simulink model "shafExPosSys"  (R2014a)
settings: Solver=ode3  StartTime=0.0  StopTime=TSIM  FixedStep=1/10  RelTol=1e-3
undefined symbols (not defined in the file): B, C, d, F, H, K, T, x1_0, x2_0, x3_0
settings Model: Creator=sqn4594  LastModifiedBy=sqn4594

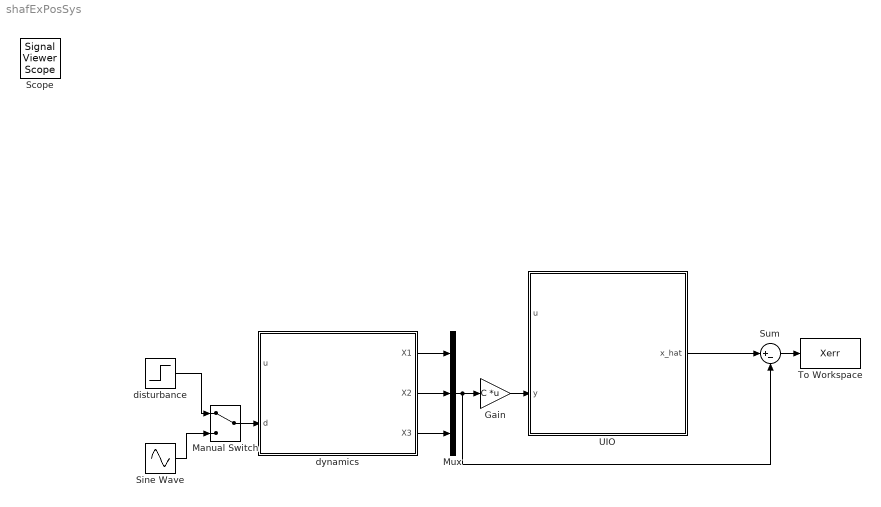
== system shafExPosSys ==
  Gain : Gain  Gain=C  Multiplication=Matrix(K*u)
  Manual Switch : ManualSwitch
  Mux : Mux  Inputs=3
  Sine Wave : Sin  Amplitude=20  Frequency=2  SampleTime=0
  Sum : Sum  Inputs=|+-
  To Workspace : ToWorkspace  VariableName=Xerr  SampleTime=-1
  UIO : Subsystem
  disturbance : Step  After=d  SampleTime=0
  dynamics : Subsystem
  Scope : SignalViewerScope  IOType=viewer  RefreshTime=0.035000
  wires:
  UIO/1(x_hat) -> Sum/1
  disturbance/1 -> Manual Switch/1
  Sine Wave/1 -> Manual Switch/2
  Sum/1 -> To Workspace/1
  dynamics/1(X1) -> Mux/1
  dynamics/2(X2) -> Mux/2
  dynamics/3(X3) -> Mux/3
  Mux/1 -> Gain/1, Sum/2
  Gain/1 -> UIO/2(y)
  Manual Switch/1 -> dynamics/2(d)

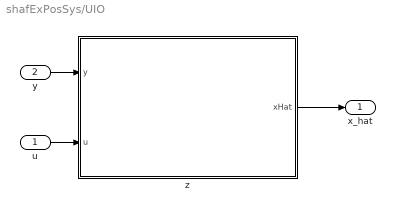
== system shafExPosSys/UIO ==
  u : Inport
  y : Inport  Port=2
  z : Subsystem
  x_hat : Outport
  wires:
  u/1 -> z/2(u)
  y/1 -> z/1(y)
  z/1(xHat) -> x_hat/1

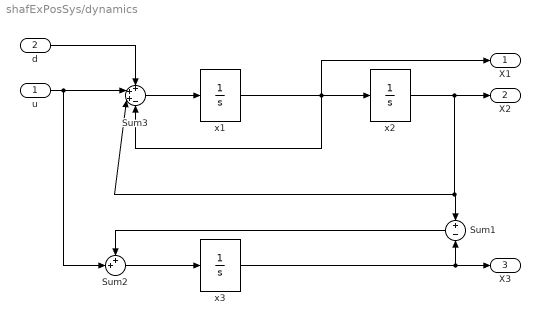
== system shafExPosSys/dynamics ==
  u : Inport
  d : Inport  Port=2
  Sum1 : Sum  Inputs=+-
  Sum2 : Sum  Inputs=++|
  Sum3 : Sum  Inputs=+++-
  x1 : Integrator  InitialCondition=x1_0
  x2 : Integrator  InitialCondition=x2_0
  x3 : Integrator  InitialCondition=x3_0
  X1 : Outport
  X2 : Outport  Port=2
  X3 : Outport  Port=3
  wires:
  Sum3/1 -> x1/1
  x1/1 -> Sum3/4, X1/1, x2/1
  x2/1 -> X2/1, Sum1/1, Sum3/3
  u/1 -> Sum2/2, Sum3/2
  d/1 -> Sum3/1
  Sum2/1 -> x3/1
  x3/1 -> Sum1/2, X3/1
  Sum1/1 -> Sum2/1

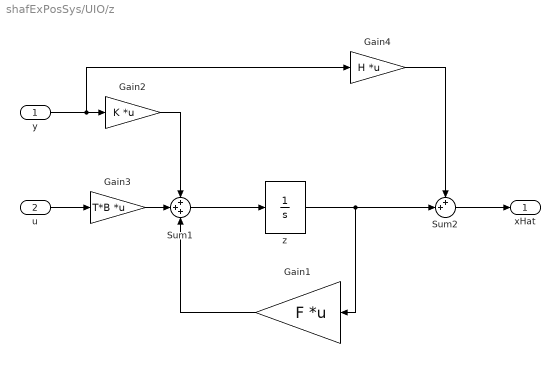
== system shafExPosSys/UIO/z ==
  y : Inport
  u : Inport  Port=2
  Gain1 : Gain  Gain=F  Multiplication=Matrix(K*u)
  Gain2 : Gain  Gain=K  Multiplication=Matrix(K*u)
  Gain3 : Gain  Gain=T*B  Multiplication=Matrix(K*u)
  Gain4 : Gain  Gain=H  Multiplication=Matrix(K*u)
  Sum1 : Sum  Inputs=+++
  Sum2 : Sum  Inputs=++|
  z : Integrator  InitialCondition=x1_0
  xHat : Outport
  wires:
  z/1 -> Sum2/2, Gain1/1
  Sum1/1 -> z/1
  Gain2/1 -> Sum1/1
  u/1 -> Gain3/1
  Gain1/1 -> Sum1/3
  Gain3/1 -> Sum1/2
  Gain4/1 -> Sum2/1
  y/1 -> Gain4/1, Gain2/1
  Sum2/1 -> xHat/1
